simulink model "Instr1_Q3cd"  (R2022b)
settings: Solver=VariableStepAuto  StartTime=0.0  StopTime=50.0  RelTol=1e-3
values from neighbouring files (symbols this model uses):
  A = [-1 0; 1 -1]    [Instr1_Q3ab.m]
  B = [1;0]    [Instr1_Q3ab.m]
  C = [0 2]    [Instr1_Q3ab.m]
  D = 0    [Instr1_Q3ab.m]
  x0 = [4,2]    [Instr1_Q3ab.m]
settings Model: Creator=maicoengelaar  LastModifiedBy=maicoengelaar

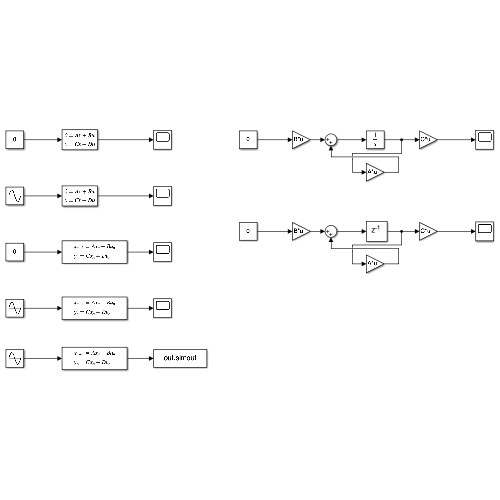
[thumbnail: Simulink's stored preview of the top-level diagram]
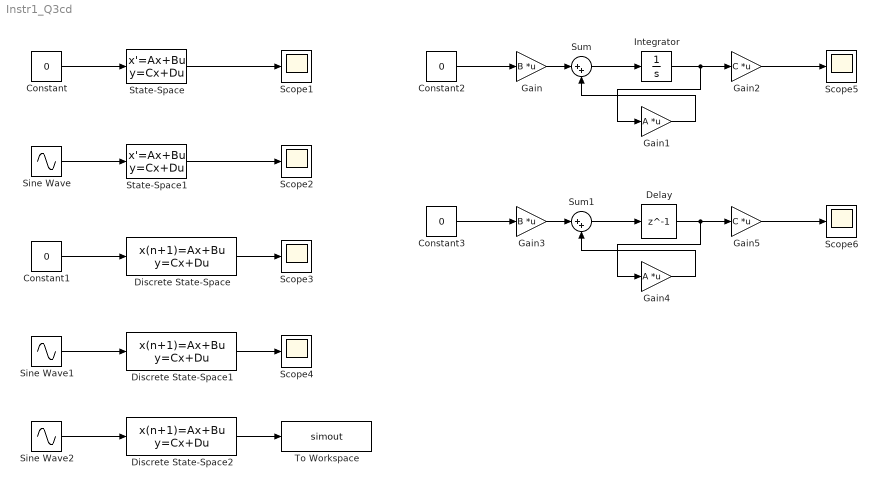
== system Instr1_Q3cd ==
  Constant : Constant  Value=0
  Constant1 : Constant  Value=0
  Constant2 : Constant  Value=0  SampleTime=1
  Constant3 : Constant  Value=0
  Delay : Delay  DelayLength=1  InitialCondition=x0
  Discrete State-Space : DiscreteStateSpace  A=A  B=B  C=C  D=D  InitialCondition=x0  SampleTime=-1
  Discrete State-Space1 : DiscreteStateSpace  A=A  B=B  C=C  D=D  InitialCondition=x0  SampleTime=-1
  Discrete State-Space2 : DiscreteStateSpace  A=A  B=B  C=C  D=D  InitialCondition=x0  SampleTime=-1
  Gain : Gain  Gain=B  Multiplication=Matrix(K*u)
  Gain1 : Gain  Gain=A  Multiplication=Matrix(K*u)
  Gain2 : Gain  Gain=C  Multiplication=Matrix(K*u)
  Gain3 : Gain  Gain=B  Multiplication=Matrix(K*u)
  Gain4 : Gain  Gain=A  Multiplication=Matrix(K*u)
  Gain5 : Gain  Gain=C  Multiplication=Matrix(K*u)
  Integrator : Integrator  InitialCondition=x0
  Scope{1..6} (6 alike) : Scope
  Sine Wave : Sin  SampleTime=0
  Sine Wave1 : Sin  SampleTime=0
  Sine Wave2 : Sin  SampleTime=0
  State-Space : StateSpace  A=A  B=B  C=C  D=D  InitialCondition=x0
  State-Space1 : StateSpace  A=A  B=B  C=C  D=D  InitialCondition=x0
  Sum : Sum  Inputs=|++
  Sum1 : Sum  Inputs=|++
  To Workspace : ToWorkspace  VariableName=simout  SaveFormat=Timeseries  SampleTime=-1
  wires:
  Constant/1 -> State-Space/1
  State-Space/1 -> Scope1/1
  Sine Wave/1 -> State-Space1/1
  State-Space1/1 -> Scope2/1
  Constant1/1 -> Discrete State-Space/1
  Sine Wave1/1 -> Discrete State-Space1/1
  Discrete State-Space/1 -> Scope3/1
  Discrete State-Space1/1 -> Scope4/1
  Sine Wave2/1 -> Discrete State-Space2/1
  Discrete State-Space2/1 -> To Workspace/1
  Constant2/1 -> Gain/1
  Gain/1 -> Sum/1
  Integrator/1 -> Gain2/1, Gain1/1
  Sum/1 -> Integrator/1
  Gain1/1 -> Sum/2
  Gain2/1 -> Scope5/1
  Constant3/1 -> Gain3/1
  Sum1/1 -> Delay/1
  Gain3/1 -> Sum1/1
  Delay/1 -> Gain5/1, Gain4/1
  Gain4/1 -> Sum1/2
  Gain5/1 -> Scope6/1
